simulink model "imu"  (R2023a)
settings: Solver=ode4  StartTime=0.0  StopTime=10.0  FixedStep=dt  RelTol=1e-3
settings Model: Creator=ndelurgio  LastModifiedBy=ndelurgio

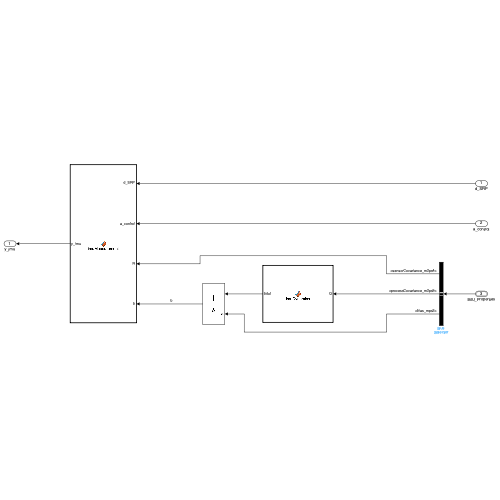
[thumbnail: Simulink's stored preview of the top-level diagram]
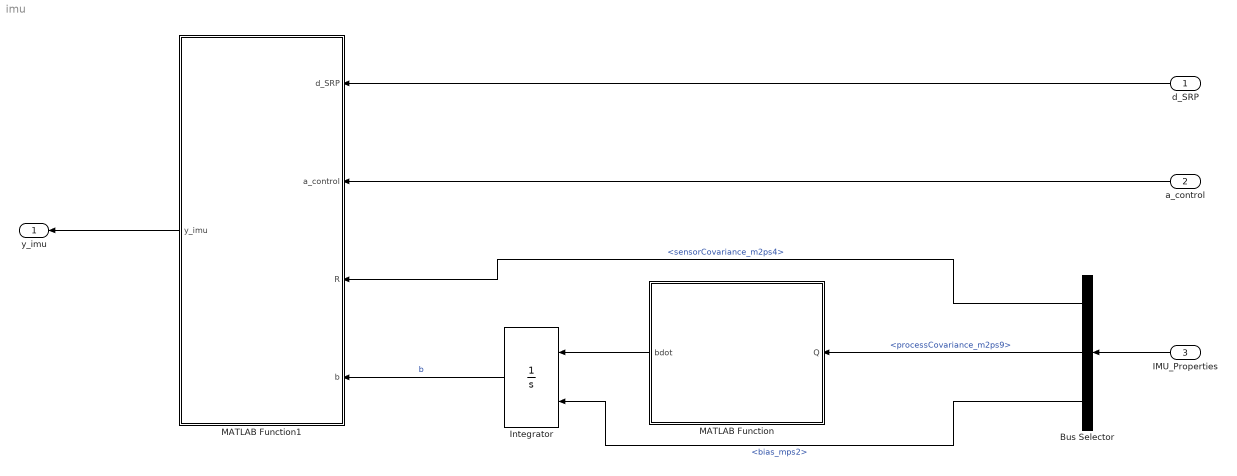
== system imu ==
  d_SRP : Inport
  a_control : Inport  Port=2
  IMU_Properties : Inport  Port=3  OutDataTypeStr=Bus: imu
  Bus Selector : BusSelector  OutputSignals=sensorCovariance_m2ps4,processCovariance_m2ps9,bias_mps2
  Integrator : Integrator  InitialConditionSource=external
  MATLAB Function : MATLAB Function  TreatAsAtomicUnit=on
  MATLAB Function1 : MATLAB Function  TreatAsAtomicUnit=on
  y_imu : Outport
  wires:
  IMU_Properties/1 -> Bus Selector/1
  Bus Selector/2 -> MATLAB Function/1(Q)  "<processCovariance_m2ps9>"
  Bus Selector/3 -> Integrator/2  "<bias_mps2>"
  MATLAB Function/1(bdot) -> Integrator/1
  Integrator/1 -> MATLAB Function1/4(b)  "b"
  Bus Selector/1 -> MATLAB Function1/3(R)  "<sensorCovariance_m2ps4>"
  a_control/1 -> MATLAB Function1/2(a_control)
  d_SRP/1 -> MATLAB Function1/1(d_SRP)
  MATLAB Function1/1(y_imu) -> y_imu/1

== matlab function imu/MATLAB Function1 ==
  data: d_SRP input; y_imu output; a_control input; R input; b input
function y_imu = imuMeasurement(d_SRP,a_control,R,b)

y_imu = imuMeasurement(d_SRP,a_control,b,R);

end

== matlab function imu/MATLAB Function ==
  data: Q input; bdot output
function bdot = imuDynamics(Q)

bdot = imuDynamics(Q);

end
